simulink model "VelocityController"  (R2017b)
settings: Solver=VariableStepAuto  StartTime=0.0  StopTime=105  RelTol=1e-3
settings Model: Creator=David Zhou  LastModifiedBy=David Zhou
settings SolverCC: AlgebraicLoopSolver=LineSearch

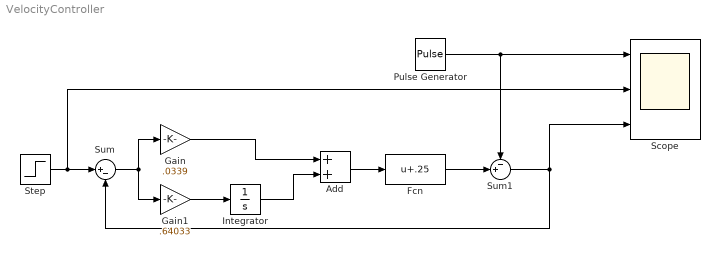
== system VelocityController ==
  Add : Sum
  Fcn : Fcn  Expr=u+.25
  Gain : Gain  Gain=.0339
  Gain1 : Gain  Gain=.64033
  Integrator : Integrator
  Pulse Generator : DiscretePulseGenerator  PulseType=Time based  Period=40  PulseWidth=50  PhaseDelay=10
  Scope : Scope  NumInputPorts=3
  Step : Step  Time=0  After=10  SampleTime=0
  Sum : Sum  Inputs=|+-
  Sum1 : Sum  Inputs=-+|
  wires:
  Sum/1 -> Gain1/1, Gain/1
  Gain1/1 -> Integrator/1
  Integrator/1 -> Add/2
  Gain/1 -> Add/1
  Add/1 -> Fcn/1
  Fcn/1 -> Sum1/2
  Sum1/1 -> Sum/2, Scope/3
  Pulse Generator/1 -> Sum1/1, Scope/1
  Step/1 -> Scope/2, Sum/1
